simulink model "Vehicle_Dynamics_Model"  (R2023b)
settings: Solver=VariableStepAuto  StartTime=0.0  StopTime=10.0  RelTol=1e-3
settings Model: Creator=Acer  LastModifiedBy=Acer

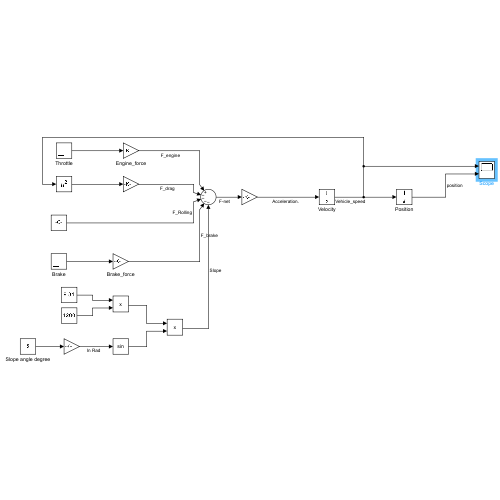
[thumbnail: Simulink's stored preview of the top-level diagram]
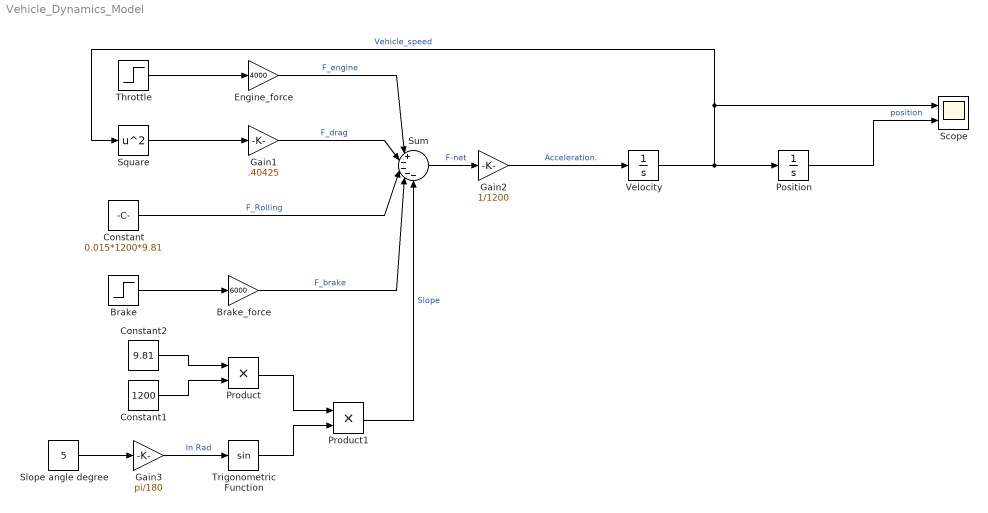
== system Vehicle_Dynamics_Model ==
  Brake : Step  Time=5  After=0.5  SampleTime=0
  Brake_force : Gain  Gain=6000
  Constant : Constant  Value=0.015*1200*9.81
  Constant1 : Constant  Value=1200
  Constant2 : Constant  Value=9.81
  Engine_force : Gain  Gain=4000
  Gain1 : Gain  Gain=.40425
  Gain2 : Gain  Gain=1/1200
  Gain3 : Gain  Gain=pi/180
  Position : Integrator
  Product : Product
  Product1 : Product
  Scope : Scope  NumInputPorts=2
  Slope angle degree : Constant  Value=5
  Square : Math  Operator=square
  Sum : Sum  Inputs=|+----
  Throttle : Step  After=.8  SampleTime=0
  Trigonometric Function : Trigonometry
  Velocity : Integrator
  wires:
  Throttle/1 -> Engine_force/1
  Gain1/1 -> Sum/2  "F_drag"
  Sum/1 -> Gain2/1  "F-net"
  Engine_force/1 -> Sum/1  "F_engine"
  Constant/1 -> Sum/3  "F_Rolling"
  Gain2/1 -> Velocity/1  "Acceleration."
  Velocity/1 -> Scope/1, Square/1, Position/1  "Vehicle_speed"
  Square/1 -> Gain1/1
  Brake/1 -> Brake_force/1
  Brake_force/1 -> Sum/4  "F_brake"
  Slope angle degree/1 -> Gain3/1
  Gain3/1 -> Trigonometric Function/1  "In Rad"
  Constant2/1 -> Product/1
  Constant1/1 -> Product/2
  Trigonometric Function/1 -> Product1/2
  Product/1 -> Product1/1
  Product1/1 -> Sum/5  "Slope"
  Position/1 -> Scope/2  "position"
